simulink model "Disturbance"  (R2016a)
settings: Solver=VariableStepAuto  StartTime=0.0  StopTime=10.0  RelTol=1e-3
settings Model: Creator=VAIO  LastModifiedBy=VAIO

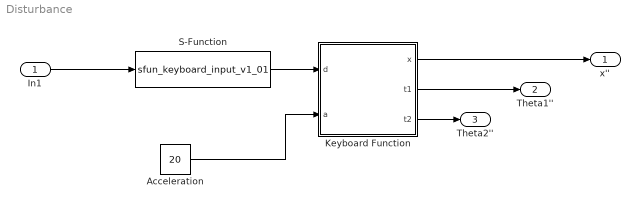
== system Disturbance ==
  In1 : Inport
  Acceleration : Constant  Value=20
  Keyboard Function : MATLAB Function  TreatAsAtomicUnit=on
  S-Function : S-Function  FunctionName=sfun_keyboard_input_v1_01  Parameters=0.01  SFunctionDeploymentMode=off  EnableBusSupport=off
  x'' : Outport
  Theta1'' : Outport  Port=2
  Theta2'' : Outport  Port=3
  wires:
  S-Function/1 -> Keyboard Function/1(d)
  Acceleration/1 -> Keyboard Function/2(a)
  In1/1 -> S-Function/1
  Keyboard Function/3(t2) -> Theta2''/1
  Keyboard Function/2(t1) -> Theta1''/1
  Keyboard Function/1(x) -> x''/1

== matlab function Disturbance/Keyboard Function ==
  data: d input; x output; a input; t1 output; t2 output
function [x,t1,t2] = fcn(d,a)

if d==28
    x=-1*a;
elseif d==29
    x=1*a;
else
    x=0;
end

if d==97
    t1=1*a;
elseif d==100
    t1=-1*a;
else
    t1=0;
end

if d==113
    t2=1*a;
elseif d==101
    t2=-1*a;
else
    t2=0;
end
